simulink model "laboratory3no1"  (R2023b)
settings: Solver=VariableStepAuto  StartTime=0.0  StopTime=10.0  RelTol=1e-3
settings Model: Creator=Emanuel  LastModifiedBy=Emanuel

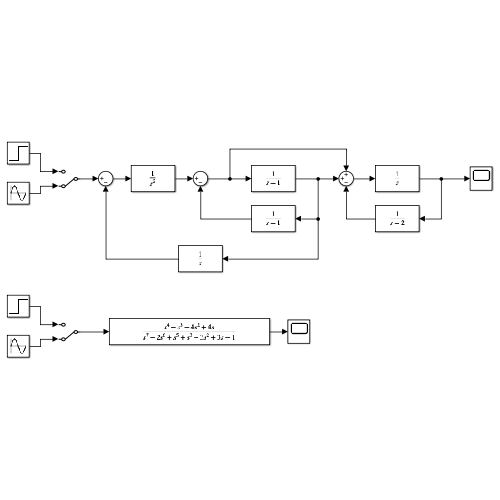
[thumbnail: Simulink's stored preview of the top-level diagram]
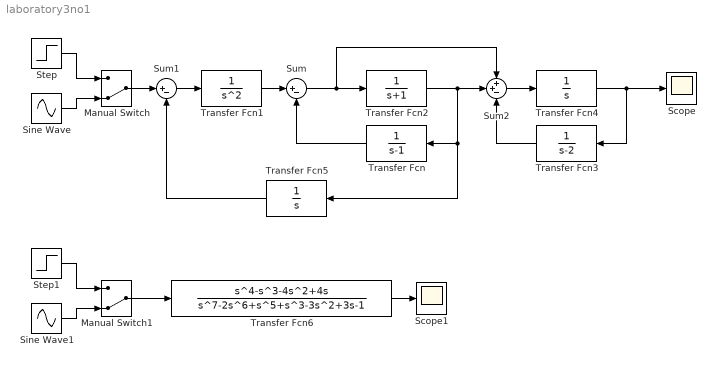
== system laboratory3no1 ==
  Manual Switch : ManualSwitch  CurrentSetting=0
  Manual Switch1 : ManualSwitch  CurrentSetting=0
  Scope : Scope
  Scope1 : Scope
  Sine Wave : Sin  SampleTime=0
  Sine Wave1 : Sin  SampleTime=0
  Step : Step  SampleTime=0
  Step1 : Step  SampleTime=0
  Sum : Sum  Inputs=|+-
  Sum1 : Sum  Inputs=|+-
  Sum2 : Sum  Inputs=++-
  Transfer Fcn : TransferFcn  Denominator=[1 -1]
  Transfer Fcn1 : TransferFcn  Denominator=[1 0 0]
  Transfer Fcn2 : TransferFcn  Denominator=[1 1]
  Transfer Fcn3 : TransferFcn  Denominator=[1 -2]
  Transfer Fcn4 : TransferFcn  Denominator=[1 0]
  Transfer Fcn5 : TransferFcn  Denominator=[1 0]
  Transfer Fcn6 : TransferFcn  Numerator=[1 -1 -4 4 0]  Denominator=[1 -2 1 0 1 -3 3 -1]
  wires:
  Transfer Fcn6/1 -> Scope1/1
  Manual Switch1/1 -> Transfer Fcn6/1
  Sine Wave1/1 -> Manual Switch1/2
  Transfer Fcn/1 -> Sum/2
  Transfer Fcn3/1 -> Sum2/3
  Transfer Fcn5/1 -> Sum1/2
  Sine Wave/1 -> Manual Switch/2
  Sum1/1 -> Transfer Fcn1/1
  Step/1 -> Manual Switch/1
  Manual Switch/1 -> Sum1/1
  Transfer Fcn4/1 -> Scope/1, Transfer Fcn3/1
  Sum/1 -> Transfer Fcn2/1, Sum2/1
  Transfer Fcn1/1 -> Sum/1
  Transfer Fcn2/1 -> Sum2/2, Transfer Fcn/1, Transfer Fcn5/1
  Step1/1 -> Manual Switch1/1
  Sum2/1 -> Transfer Fcn4/1
